simulink model "testSimulink"  (R2022b)
settings: Solver=FixedStepAuto  StartTime=0.0  StopTime=10.0  RelTol=1e-3
libraries: androidadvancedlib x2, androidaudiovideolib x1
settings Model: Creator=xuezh  LastModifiedBy=xuezh
settings OptimizationCC: EnhancedBackFolding=on  PassReuseOutputArgsAs=Individual arguments  ZeroExternalMemoryAtStartup=off  ZeroInternalMemoryAtStartup=off  MaxStackSize=64  OptimizeBlockOrder=speed  DifferentSizesBufferReuse=on  OptimizationCustomize=off  EfficientTunableParamExpr=on
settings DebuggingCC: ParameterTunabilityLossMsg=error
settings HardwareCC: ProdBitPerPointer=32  ProdBitPerSizeT=32  ProdBitPerPtrDiffT=32  ProdLargestAtomicInteger=Long  ProdLargestAtomicFloat=Double  ProdWordSize=32  ProdHWDeviceType=ARM Compatible->ARM Cortex
settings SFSimCC: MATLABDynamicMemAlloc=off
settings RTWCC: Description=Embedded Coder  SystemTargetFile=ert.tlc  HardwareBoard=Android Device  TLCOptions="-aInlineSetEventsForThisBaseRateFcn=TLC_FALSE -aSuppressMultiTaskScheduler=TLC_FALSE  -aRateBasedStepFcn=0"  TemplateMakefile=ert_default_tmf  RTWVerbose=off  Toolchain=Android SDK/NDK Tools
settings CodeAppCC: ForceParamTrailComments=on  IgnoreCustomStorageClasses=off  OperatorAnnotations=on  SimulinkDataObjDesc=on  SFDataObjDesc=on  InsertBlockDesc=on

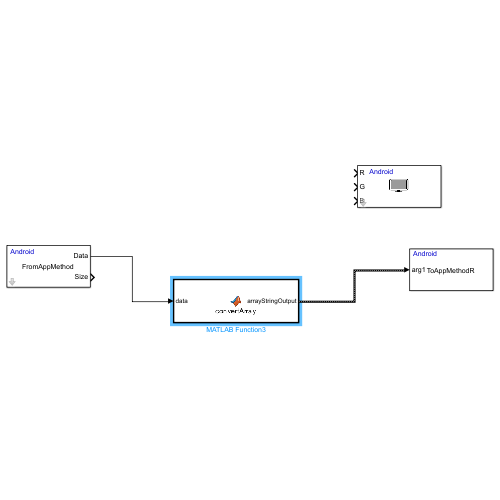
[thumbnail: Simulink's stored preview of the top-level diagram]
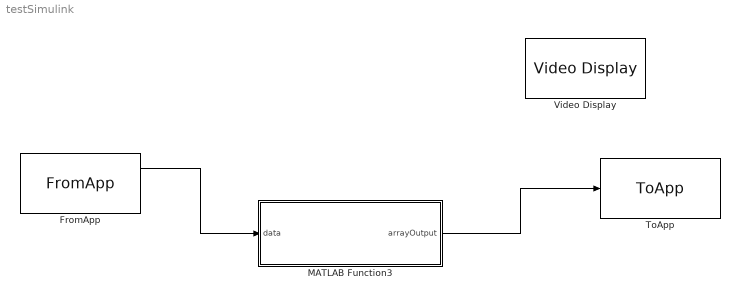
== system testSimulink ==
  FromApp : androidadvancedlib/FromApp  FunctionName=FromAppMethod  DataType=double  DataSize=268435455  SampleTime=0.1  BlockPlatform=Android  MaskFuncName='FromAppMethod'
  MATLAB Function3 : MATLAB Function  TreatAsAtomicUnit=on
  ToApp : androidadvancedlib/ToApp  FunctionName=ToAppMethodR  NumInputs=1
  Video Display : androidaudiovideolib/Video Display  BlockPlatform=Android
  wires:
  FromApp/1 -> MATLAB Function3/1(data)
  MATLAB Function3/1(arrayOutput) -> ToApp/1

== matlab function testSimulink/MATLAB Function3 ==
  data: data input; arrayOutput output
function arrayOutput = convertArray(data) %   For,string
% function [r,g,b] = convertArray(data)
%% data = [N x 1] array 
%% arrayOutput = [1 x N] array
imgLength = data(1);
width  = data(2);
%arraySize = size(data);
sizeOfArray = imgLength * width * 3;
sizeOfImage = imgLength * width;
hdrArray = zeros(1, 1,3);
arrayToAndroid = zeros(1,numel(sizeOfArray));
if numel(data) < 134217728
    newData = data(3:sizeOfArray+2);
    if sizeOfImage < 44739242
        hdrArray = zeros(imgLength, width,3);
        if numel(newData) == sizeOfArray && sizeOfArray ~= 0
            hdrArray = reshape(newData,[imgLength, width,3]);
            ldrImgArray = DCA_TMO(hdrArray);
            arrayToAndroid = reshape(ldrImgArray,1, numel(ldrImgArray));
        end
    end
end

if numel(arrayToAndroid) < 3
    arrayOutput = [9 9 9];
else
    arrayOutput = arrayToAndroid;
end
end


function ldrImg = DCA_TMO(hdrImg)

%% set parameters
K = 55;

%% pre-processing
% [N, M, C] = size(hdrImg);
maxhdr = MaxQuart(hdrImg(:), 0.99);
minhdr = MaxQuart(hdrImg(:), 0.01);
hdrImg(hdrImg>maxhdr) = maxhdr;
hdrImg(hdrImg<minhdr) = minhdr;

%% tone map using clustering method
hdrLum = 0.2126 * hdrImg(:,:,1) + 0.7152 * hdrImg(:,:,2) + 0.0722 * hdrImg(:,:,3);
hdrLum1 = hdrLum./max(hdrImg(:));
hdrPQ = ((107/128 + 2413/128*hdrLum1.^(1305/8192)) ./ (1 + 2392/128*hdrLum1.^(1305/8192))) .^ (2523/32);
[labels, ~, ~] = quantizeNL_float(hdrPQ, K, hdrLum);

%% local enhancemant using DoG
sigmaC = 0.5;
sigmaS = 0.8;
window = 9;
gfilterC = fspecial('gaussian', window, sigmaC);
gfilterS = fspecial('gaussian', window, sigmaS);
DoGfilter = gfilterC - gfilterS;
hdrPQnor = 255 .* (hdrPQ - min(hdrPQ(:))) ./ (max(hdrPQ(:)) - min(hdrPQ(:))) + 1;
hdrPQnor = hdrPQnor .* 0.35 + labels .* 0.65;
labels_DoG = labels + 3.0*imfilter(hdrPQnor, DoGfilter, 'replicate');

%% color restoration
s1 = (labels_DoG - min(labels_DoG(:))) ./ (max(labels_DoG(:)) - min(labels_DoG(:)));
s = 1 - atan(s1);
s = min(s, 0.5);
ldrImg_DoG = (hdrImg ./ hdrLum).^s .* labels_DoG;
maxx = MaxQuart(ldrImg_DoG(:), 0.99);
minn = MaxQuart(ldrImg_DoG(:), 0.01);
if maxx<255
    if max(ldrImg_DoG(:))<255
        maxx = max(ldrImg_DoG(:));
    else
        maxx = 255;
    end
end
if minn>0
    if min(ldrImg_DoG(:))>0
        minn = min(ldrImg_DoG(:));
    else
        minn = 0;
    end
end
ldrImg_DoG(ldrImg_DoG>maxx) = maxx;
ldrImg_DoG(ldrImg_DoG<minn) = minn;
ldrImg = 255.* ((ldrImg_DoG - minn) ./ (maxx - minn));
end

function [ labels, mdata, edges ] = quantizeNL_float( y, nclust, lum )
% y is input data
% nclust is the number of clusters or quantization levels. If you want to
% quantize data with b bits then nclust <= 2^b (256 if b=8)
% labels are the quantization intervals in [1, nclust] range assigned to y
% mdata is the mean value of each cluster

lum = double(lum);
lum0 = lum;
lum = reshape(lum, 1, numel(lum));
lum = sort(lum);

y = double(y);
y = reshape(y, 1, numel(y));
y = sort(y);

edges= ones(1,56); % Added initialization to ensure left and right data matches
errors= ones(1,55); % Added initialization to ensure left and right data matches
edges = [0,numel(y)];
errors = sum((y-mean(y)).^2);

s_data = cumsum(y);
ss_data = cumsum(y.^2);

for i = 1 : nclust-1
    [~,idx] = max(errors);
    k = edges(idx); n = edges(idx+1)-k;
    sn = s_data(k+n); 
    if(k>=1) 
        sn = sn - s_data(k); 
    end
    ssn = ss_data(k+n); 
    if(k>=1) 
        ssn = ssn - ss_data(k); 
    end
    d = 2; m = floor(n/d);
    while(1)
        sm = s_data(k+m); 
        if(k>=1) 
            sm = sm - s_data(k); 
        end
        ssm = ss_data(k+m); 
        if(k>=1) 
            ssm = ssm - ss_data(k); 
        end
        e1 = ssm-sm^2/m;
        e2 = ssn - ssm - (sn - sm)^2/(n-m);
        d = 2 * d;
        if(abs(e1-e2) < 0.001 || d >= n)
            lum1 = median(lum(k+1:k+m)); lum2 = median(lum(k+m+1:k+n));
            delta1 = 10.^tvi(log10(lum1)); delta2 = 10.^tvi(log10(lum2));
            [~, lum_loc] = min(abs(delta1./(delta1+delta2) .* (lum(k+n)-lum(k+1)) + lum(k+1) - lum(k+1:k+n)));
            m = lum_loc;
            sm = s_data(k+m); 
            if(k>=1) 
                sm = sm - s_data(k); 
            end
            ssm = ss_data(k+m); 
            if(k>=1) 
                ssm = ssm - ss_data(k); 
            end
            e1 = ssm-sm^2/m;
            e2 = ssn - ssm - (sn - sm)^2/(n-m);
            
            edges = [edges(1:idx),k+m,edges(idx+1:end)];
            errors = [errors(1:idx-1),e1,e2,errors(idx+1:end)];
            break;
        else
            if(e1 > e2) 
                m = m-floor(n/d); 
            elseif(e1 < e2) 
                m = m+floor(n/d); 
            end
        end
    end
end

mdata = zeros(1, nclust);
mdata(1) = min(lum0(:));
mdata(end) = max(lum0(:));
for i=2:nclust-1
    if lum(edges(i))==lum(edges(i+1))
        ind = (lum0==lum(edges(i)));
        mdata(i) = mean(lum0(ind))+eps*i;
    else
        ind = (lum0>lum(edges(i)) & lum0<=lum(edges(i+1)));
        mdata(i) = mean(lum0(ind));
    end
end

labels_mdata = linspace(1, 256, nclust);
labels = interp1(mdata, labels_mdata, lum0, 'linear');

end

function ret = MaxQuart(matrix, percentile)
%
%
%       ret = MaxQuart(matrix, percentile)
%
%
%       Input:
%           -matrix: a matrix
%           -percentile: a value in the range [0,1]
%
%       Output:
%           -ret: the percentile of the input matrix
%
%     Copyright (C) 2011-2015  Francesco Banterle
% 
%     This program is free software: you can redistribute it and/or modify
%     it under the terms of the GNU General Public License as published by
%     the Free Software Foundation, either version 3 of the License, or
%     (at your option) any later version.
% 
%     This program is distributed in the hope that it will be useful,
%     but WITHOUT ANY WARRANTY; without even the implied warranty of
%     MERCHANTABILITY or FITNESS FOR A PARTICULAR PURPOSE.  See the
%     GNU General Public License for more details.
% 
%     You should have received a copy of the GNU General Public License
%     along with this program.  If not, see <http://www.gnu.org/licenses/>.
%

if(percentile > 1.0)
    percentile = 1.0;
end

if(percentile < 0.0)
    percentile = 0.0;
end

[n, m] = size(matrix);

matrix = sort(reshape(matrix, n * m, 1));
index = round(n * m * percentile);
index = max([index 1]);
ret = matrix(index);

end

function threshold = tvi(intensity)
%---------------------------------------
% The output is the sensitivity of HVS measured as just noticeable
% difference in the ambient intensity defined by the input parameter.
%
% intensity: real luminance in log10 domain
% threshold: in log10 domain, delta(lum)=10.^(threshold)

threshold = zeros(size(intensity));

idx = find(intensity < -3.94);
threshold (idx) = -2.86;

idx = find(intensity >= -3.94 & intensity < -1.44);
threshold (idx) = (0.405 * intensity(idx) + 1.6) .^ 2.18 - 2.86;

idx = find(intensity >= -1.44 & intensity < -0.0184);
threshold (idx) = intensity(idx) - 0.395;

idx = find(intensity >= -0.0184 & intensity < 1.9);
threshold(idx) = (0.249 * intensity(idx) + 0.65) .^ 2.7 - 0.72;

idx = find(intensity >= 1.9);
threshold (idx) = intensity(idx) - 1.255;

threshold = threshold - 0.95;
end
